simulink model "power_dcmotor"  (R2016b)
settings: Solver=ode23tb  StartTime=0.0  StopTime=10  RelTol=1e-4
libraries: powerlib x17, powerlib_meascontrol x1, simulink x1
Description:
  | Copyright 2008-2016 The MathWorks, Inc.
settings Model: ExtModeTrigMode=oneshot  ExtModeArmWhenConnect=off  ExtModeAutoUpdateStatusClock=off  Creator=MathWorks  LastModifiedBy=batserve
settings SolverCC: ZeroCrossAlgorithm=Adaptive
settings DataIOCC: Decimation=5  FinalStateName=x50  InitialState=x50  MaxDataPoints=500000  SaveFormat=Array  SignalLoggingSaveFormat=ModelDataLogs  SaveOutput=off  TimeSaveName=t  SignalLoggingName=sigsOut
settings OptimizationCC: BlockReduction=off  BooleanDataType=off  ExpressionDepthLimit=2147483647  InitFltsAndDblsToZero=on  EfficientMapNaN2IntZero=off  LifeSpan=inf
settings DebuggingCC: UnderspecifiedInitializationDetection=Classic  MergeDetectMultiDrivingBlocksExec=none  CheckExecutionContextPreStartOutputMsg=on  CheckExecutionContextRuntimeOutputMsg=on  SignalResolutionControl=TryResolveAllWithWarning  MultiTaskDSMMsg=warning  MultiTaskCondExecSysMsg=none  SigSpecEnsureSampleTimeMsg=none  IntegerOverflowMsg=none  FcnCallInpInsideContextMsg=warning  StateNameClashWarn=warning  SFUnexpectedBacktrackingDiag=warning  SFNoUnconditionalDefaultTransitionDiag=warning  SFExecutionAtInitializationDiag=none  IntegerSaturationMsg=none
settings HardwareCC: ProdBitPerPointer=32  ProdBitPerSizeT=32  ProdBitPerPtrDiffT=32  ProdLargestAtomicFloat=None  ProdIntDivRoundTo=Undefined  ProdEndianess=Unspecified  ProdWordSize=32  ProdHWDeviceType=32-bit Generic  TargetUnknown=on
settings ModelReferenceCC: PropagateSignalLabelsOutOfModel=off
settings GRTTargetCC: TargetLangStandard=C89/C90 (ANSI)  GeneratePreprocessorConditionals=Disable all  CombineOutputUpdateFcns=off  GRTInterface=on
settings ConfigComp: CovMetricSettings=dw  CovHtmlReporting=on  CovSaveCumulativeToWorkspaceVar=on  CovSaveSingleToWorkspaceVar=on  CovExternalEMLEnable=off  CovSFcnEnable=off

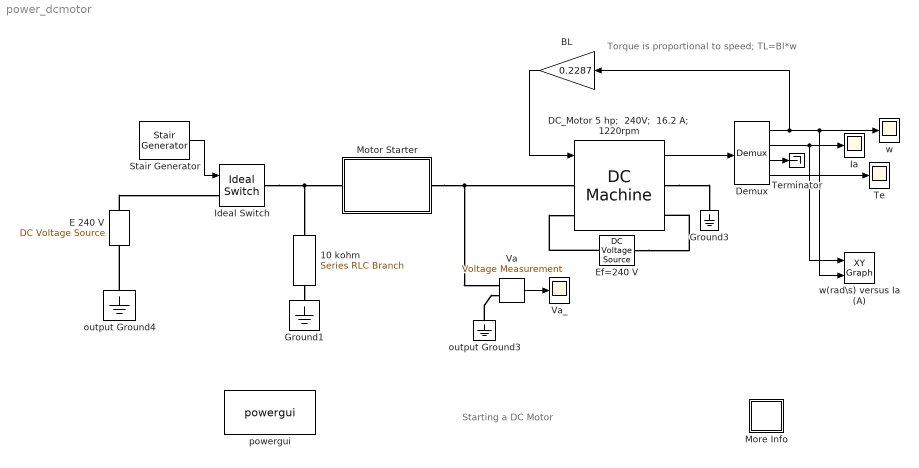
== system power_dcmotor ==
  note: Starting a DC Motor
  note: Torque is proportional to speed; TL=Bl*w
  10 kohm : powerlib/Elements/Series RLC Branch  LConnTagsString=__new0  RConnTagsString=__new0  BranchType=R  Resistance=1e4  Inductance=[]  SetiL0=off  InitialCurrent=0  Capacitance=[]  Setx0=off  InitialVoltage=0  Measurements=None
  BL : Gain  Gain=0.2287  SaturateOnIntegerOverflow=on  OutDataTypeStr=Inherit: Same as input  ParamDataTypeStr=Inherit: Same as input
  DC_Motor 5 hp;  240V;  16.2 A;  1220rpm : powerlib/Machines/DC Machine  PresetModel=No  MechanicalLoad=Torque TL  FieldType=Wound  ShowDetailedParameters=on  MeasurementBus=off  RLa="[ 0.6  0.012]"  RLf="[ 240  120]"  Laf=1.8  MachineConstant=Torque constant (N.m/A)  Ke=1.8  Kt=1.8  J=1  Bm=0  Tf=0  w0=1  Ifinit=1  TsPowergui=0  TsBlock=-1
      settings: AttributesFormatString=\n
  Demux : Demux
  E 240 V : powerlib/Electrical Sources/DC Voltage Source  Description=source block  Amplitude=240  Measurements=None
      settings: AttributesFormatString=\n
  Ef=240 V : powerlib/Electrical Sources/DC Voltage Source  Description=source block  Amplitude=240  Measurements=None
      settings: AttributesFormatString=\n
  Ground1 : powerlib/Elements/Ground  LConnTagsString=a
  Ground3 : powerlib/Elements/Ground  LConnTagsString=a
  Ia : Scope
  Ideal Switch : powerlib/Power Electronics/Ideal Switch  Ron=1e-4  Lon=10e-6  IC=0  Rs=inf  Cs=0  Measurements=off
      settings: AttributesFormatString=\n
  More Info : Subsystem
      settings: OpenFcn=showdemo(bdroot(gcb))
      mask Display: disp('?')
  "Motor Starter " : Subsystem
      mask Display: disp('3 step\n\nstarter')
  Stair Generator : powerlib_meascontrol/Pulse & Signal Generators/Stair Generator  t=[0 0.5 ]  e=[0 1 ]  Ts=0
  Te : Scope
  Terminator : Terminator
  Va : powerlib/Measurements/Voltage Measurement  Tag=PoWeRsYsTeMmEaSuReMeNt  PhasorSimulation=off  OutputType=Magnitude  PSBequivalent=0
  Va_ : Scope
  output Ground3 : powerlib/Elements/Ground  LConnTagsString=a
  output Ground4 : powerlib/Elements/Ground  LConnTagsString=a
  powergui : powerlib/powergui  Priority=2  SimulationMode=Continuous  SolverType=Tustin  SampleTime=0  frequency=60  SPID=on  DisableSnubberDevices=on  DisableRonSwitches=off  DisableVfSwitches=off  SwTol=0  DisplayEquations=off  Interpol=off  ExternalGateDelay=off  methode=off  Ts=0  FunctionMessages=off  echomessages=off  HookPort=off  EnableUseOfTLC=off  x0status=blocks  frequencyindice=0  Pbase=100e6  ErrMax=1e-4  Iterations=50  UnitsV=kV  UnitsW=MW  buscounter=0  RestoreLinks=warning  ResistiveCurrentMeasurement=off  Frange=logspace(0,3,50)  Ylog=off  Xlog=off  ShowGrid=off  save=off  variable=ZData  structure=0  ZoomFFT=on  StartTime=0.0  cycles=1  DisplayStyle=off  fundamental=60  FreqAxis=off  MaxFrequency=1000  frequencyindicesteady=1  RmsSteady=1  display=off
  w : Scope
  w(rad\s) versus Ia (A) : simulink/Sinks/XY Graph  xmin=0  xmax=40  ymin=0  ymax=140  st=-1
  wires:
  Demux/4 -> Te/1
  Demux/1 -> BL/1, w/1, w(rad\s) versus Ia (A)/2
  Demux/2 -> Ia/1, w(rad\s) versus Ia (A)/1
  Demux/3 -> Terminator/1
  Stair Generator/1 -> Ideal Switch/1
  Va/1 -> Va_/1
  DC_Motor 5 hp;  240V;  16.2 A;  1220rpm/1 -> Demux/1
  BL/1 -> DC_Motor 5 hp;  240V;  16.2 A;  1220rpm/1
  connections:
  output Ground4/LConn1 -- E 240 V/LConn1
  10 kohm/RConn1 -- Ground1/LConn1
  Ideal Switch/RConn1 -- 10 kohm/LConn1 -- "Motor Starter "/LConn1
  E 240 V/RConn1 -- Ideal Switch/LConn1
  "Motor Starter "/RConn1 -- Va/LConn1 -- DC_Motor 5 hp;  240V;  16.2 A;  1220rpm/LConn1
  DC_Motor 5 hp;  240V;  16.2 A;  1220rpm/RConn1 -- Ground3/LConn1
  output Ground3/LConn1 -- Va/LConn2
  Ef=240 V/LConn1 -- DC_Motor 5 hp;  240V;  16.2 A;  1220rpm/RConn2
  Ef=240 V/RConn1 -- DC_Motor 5 hp;  240V;  16.2 A;  1220rpm/LConn2

== system power_dcmotor/More Info ==

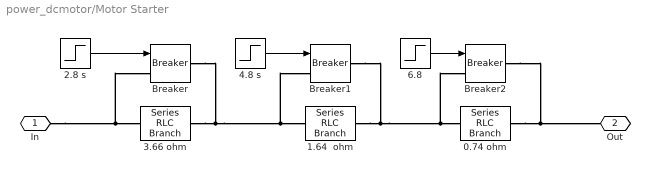
== system power_dcmotor/Motor Starter  ==
  0.74 ohm : powerlib/Elements/Series RLC Branch  LConnTagsString=__new0  RConnTagsString=__new0  BranchType=R  Resistance=0.74  Inductance=[]  SetiL0=off  InitialCurrent=0  Capacitance=[]  Setx0=off  InitialVoltage=0  Measurements=None
  1.64  ohm : powerlib/Elements/Series RLC Branch  LConnTagsString=__new0  RConnTagsString=__new0  BranchType=R  Resistance=1.64  Inductance=[]  SetiL0=off  InitialCurrent=0  Capacitance=[]  Setx0=off  InitialVoltage=0  Measurements=None
  2.8 s : Step  Time=2.8  SampleTime=0
  3.66 ohm : powerlib/Elements/Series RLC Branch  LConnTagsString=__new0  RConnTagsString=__new0  BranchType=R  Resistance=3.66  Inductance=[]  SetiL0=off  InitialCurrent=0  Capacitance=[]  Setx0=off  InitialVoltage=0  Measurements=None
  4.8 s : Step  Time=4.8  SampleTime=0
  6.8 : Step  Time=6.8  SampleTime=0
  Breaker : powerlib/Elements/Breaker  InitialState=0  SwitchingTimes="[ 4/60  5/60 ]"  External=on  BreakerResistance=0.01  SnubberResistance=inf  SnubberCapacitance=0  Measurements=None  MoreParameters=off  NoBreakLoop=off
      settings: AttributesFormatString=\n
  Breaker1 : powerlib/Elements/Breaker  InitialState=0  SwitchingTimes="[ 4/60  5/60 ]"  External=on  BreakerResistance=0.01  SnubberResistance=inf  SnubberCapacitance=0  Measurements=None  MoreParameters=off  NoBreakLoop=off
      settings: AttributesFormatString=\n
  Breaker2 : powerlib/Elements/Breaker  InitialState=0  SwitchingTimes="[ 4/60  5/60 ]"  External=on  BreakerResistance=0.01  SnubberResistance=inf  SnubberCapacitance=0  Measurements=None  MoreParameters=off  NoBreakLoop=off
      settings: AttributesFormatString=\n
  In : PMIOPort  Port=1  Side=Left
  Out : PMIOPort  Port=2  Side=Right
  wires:
  4.8 s/1 -> Breaker1/1
  6.8/1 -> Breaker2/1
  2.8 s/1 -> Breaker/1
  connections:
  In/RConn1 -- 3.66 ohm/LConn1 -- Breaker/LConn1
  3.66 ohm/RConn1 -- 1.64  ohm/LConn1 -- Breaker1/LConn1 -- Breaker/RConn1
  1.64  ohm/RConn1 -- 0.74 ohm/LConn1 -- Breaker2/LConn1 -- Breaker1/RConn1
  0.74 ohm/RConn1 -- Out/RConn1 -- Breaker2/RConn1
